simulink model "SLIPquadold"  (R2015a)
settings: Solver=ode45  StartTime=0.0  StopTime=5  MaxStep=1e-3  RelTol=1e-4  AbsTol=1e-6
values from neighbouring files (symbols this model uses):
  a0 = 68*pi/180    (= 1.18682389136)    [smm_params.m]
  dt0 = -0.3325    [SLIPquad_params.m]
  dx0 = 0.4138    [SLIPquad_params.m]    (also in SLIPrun_params.m = 3; SLIPwalk_params.m = 2.5; smm_params.m = 5)
  dy0 = 0.1683    [SLIPquad_params.m]    (also in SLIPrun_params.m = -1; SLIPwalk_params.m = 0; smm_params.m = 0)
  g = 1    [SLIPquad_params.m]    (also in SLIPrun_params.m = 9.81; SLIPwalk_params.m = 9.81; smm_params.m = 9.81)
  J = 0.6    [SLIPquad_params.m]
  k = 20    [SLIPquad_params.m]    (also in SLIPrun_params.m = 23000; SLIPwalk_params.m = 10000; smm_params.m = 20000)
  L = sqrt( (u(3)-u(1))^2 + (u(4)-u(2))^2 )    [AnimSMR.m]    (also in SLIPquad_params.m = 0.5)
  l0 = 1    [SLIPquad_params.m]    (also in SLIPrun_params.m; SLIPwalk_params.m; smm_params.m)
  m = 1    [SLIPquad_params.m]    (also in SLIPrun_params.m = 70; SLIPwalk_params.m = 70; smm_params.m = 80)
  t0 = 0.056    [SLIPquad_params.m]
  x0 = []    [AnimQUAD.m]    (also in AnimQUAD2.m; AnimSMR.m; SLIPquad_params.m = 0; SLIPrun_params.m = -l*sin(theta_th))
  xrb0 = -l0*cos(a0br) + L*cos(t0)    [SLIPquad_params.m]
  xrf0 = -l0*cos(a0fr) - L*cos(t0)    [SLIPquad_params.m]
  y0 = 1.0237    [SLIPquad_params.m]    (also in SLIPrun_params.m = sqrt(l^2 - x0^2); SLIPwalk_params.m = sqrt(l0^2 - x0^2); smm_params.m = 1)
  yrb0 = l0*sin(a0br) + L*sin(t0)    [SLIPquad_params.m]
  yrf0 = l0*sin(a0fr) - L*sin(t0)    [SLIPquad_params.m]
libraries: simulink_extras x2
settings Model: Creator=hgeyer  LastModifiedBy=Joe
settings DataIOCC: LimitDataPoints=off  SignalLoggingSaveFormat=ModelDataLogs
settings OptimizationCC: ExpressionDepthLimit=2147483647
settings DebuggingCC: UnderspecifiedInitializationDetection=Classic  MergeDetectMultiDrivingBlocksExec=none  SolverPrmCheckMsg=warning  FcnCallInpInsideContextMsg=EnableAllAsWarning  StateNameClashWarn=warning

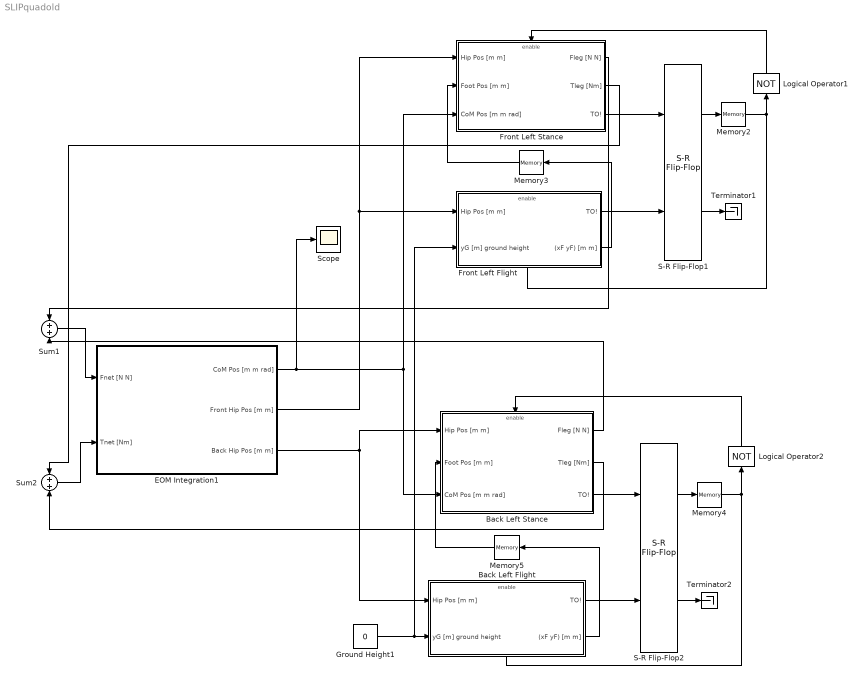
== system SLIPquadold ==
  Back Left Flight : Subsystem
  Back Left Stance : Subsystem
  EOM Integration1 : Subsystem
  Front Left Flight : Subsystem
  Front Left Stance : Subsystem
  Ground Height1 : Constant  Value=0
  Logical Operator1 : Logic  Operator=NOT  AllPortsSameDT=off  OutDataTypeStr=boolean
  Logical Operator2 : Logic  Operator=NOT  AllPortsSameDT=off  OutDataTypeStr=boolean
  Memory2 : Memory  X0=1
  Memory3 : Memory  X0=[(x0 - xrf0) (y0 - yrf0)]
  Memory4 : Memory  X0=1
  Memory5 : Memory  X0=[(x0 - xrb0) (y0 - yrb0)]
  S-R Flip-Flop1 : simulink_extras/Flip Flops/S-R Flip-Flop  initial_condition=1
  S-R Flip-Flop2 : simulink_extras/Flip Flops/S-R Flip-Flop  initial_condition=1
  Scope : Scope
  Sum1 : Sum  Inputs=+|+
  Sum2 : Sum  Inputs=+|+
  Terminator1 : Terminator
  Terminator2 : Terminator
  wires:
  Front Left Stance/3(TO!) -> S-R Flip-Flop1/1
  S-R Flip-Flop1/1 -> Memory2/1
  Front Left Flight/1(TO!) -> S-R Flip-Flop1/2
  Memory2/1 -> Front Left Flight/Enable, Logical Operator1/1
  Logical Operator1/1 -> Front Left Stance/Enable
  S-R Flip-Flop1/2 -> Terminator1/1
  Front Left Flight/2((xF yF) [m m]) -> Memory3/1
  Memory3/1 -> Front Left Stance/2(Foot Pos [m m])
  Back Left Stance/3(TO!) -> S-R Flip-Flop2/1
  S-R Flip-Flop2/1 -> Memory4/1
  Back Left Flight/1(TO!) -> S-R Flip-Flop2/2
  Memory4/1 -> Back Left Flight/Enable, Logical Operator2/1
  Logical Operator2/1 -> Back Left Stance/Enable
  S-R Flip-Flop2/2 -> Terminator2/1
  Back Left Flight/2((xF yF) [m m]) -> Memory5/1
  Memory5/1 -> Back Left Stance/2(Foot Pos [m m])
  Front Left Stance/1(Fleg [N N]) -> Sum1/1
  Back Left Stance/1(Fleg [N N]) -> Sum1/2
  Front Left Stance/2(Tleg [Nm]) -> Sum2/1
  Back Left Stance/2(Tleg [Nm]) -> Sum2/2
  Sum1/1 -> EOM Integration1/1(Fnet [N N])
  Sum2/1 -> EOM Integration1/2(Tnet [Nm])
  EOM Integration1/2(Front Hip Pos [m m]) -> Front Left Flight/1(Hip Pos [m m]), Front Left Stance/1(Hip Pos [m m])
  EOM Integration1/3(Back Hip Pos [m m]) -> Back Left Flight/1(Hip Pos [m m]), Back Left Stance/1(Hip Pos [m m])
  EOM Integration1/1(CoM Pos [m m rad]) -> Scope/1, Front Left Stance/3(CoM Pos [m m rad]), Back Left Stance/3(CoM Pos [m m rad])
  Ground Height1/1 -> Front Left Flight/2(yG [m] ground height), Back Left Flight/2(yG [m] ground height)

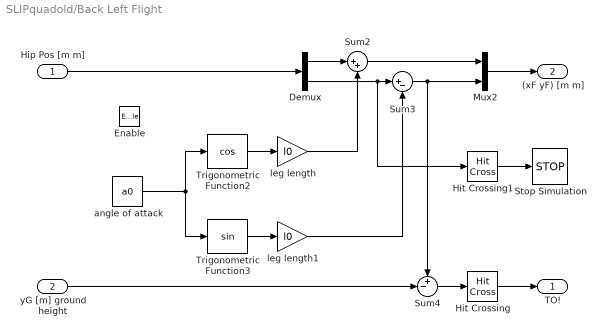
== system SLIPquadold/Back Left Flight ==
  Hip Pos [m m] : Inport
  yG [m] ground height : Inport  Port=2
  Enable : EnablePort  StatesWhenEnabling=reset
  Demux : Demux  Outputs=2
  Hit Crossing : HitCross  HitCrossingDirection=falling
  Hit Crossing1 : HitCross  HitCrossingDirection=falling
  Mux2 : Mux  Inputs=2
  Stop Simulation : Stop
  Sum2 : Sum  Inputs=|++
  Sum3 : Sum  Inputs=|+-
  Sum4 : Sum  Inputs=+-|
  Trigonometric Function2 : Trigonometry  Operator=cos
  Trigonometric Function3 : Trigonometry
  angle of attack : Constant  Value=a0
  leg length : Gain  Gain=l0
  leg length1 : Gain  Gain=l0
  TO! : Outport  OutputWhenDisabled=reset  InitialOutput=0
      settings: AttributesFormatString=%<OutputWhenDisabled>
  (xF yF) [m m] : Outport  Port=2  InitialOutput=[0 0]
      settings: AttributesFormatString=%<OutputWhenDisabled>
  wires:
  Hit Crossing/1 -> TO!/1
  Demux/2 -> Hit Crossing1/1, Sum3/1
  Demux/1 -> Sum2/1
  angle of attack/1 -> Trigonometric Function3/1, Trigonometric Function2/1
  Trigonometric Function2/1 -> leg length/1
  Trigonometric Function3/1 -> leg length1/1
  Hip Pos [m m]/1 -> Demux/1
  leg length/1 -> Sum2/2
  leg length1/1 -> Sum3/2
  Sum3/1 -> Mux2/2, Sum4/1
  Sum2/1 -> Mux2/1
  Mux2/1 -> (xF yF) [m m]/1
  yG [m] ground height/1 -> Sum4/2
  Sum4/1 -> Hit Crossing/1
  Hit Crossing1/1 -> Stop Simulation/1

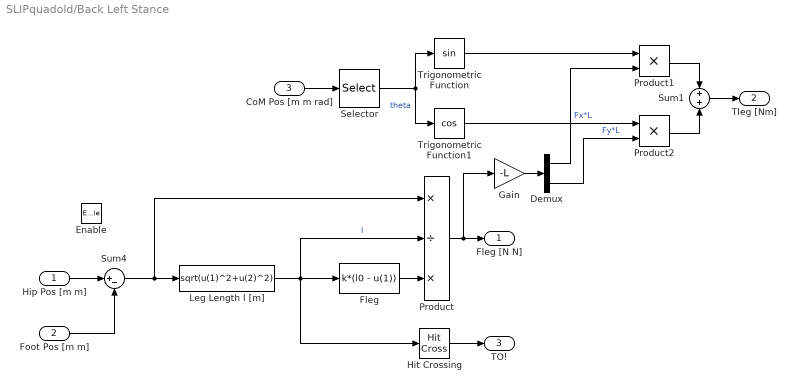
== system SLIPquadold/Back Left Stance ==
  Hip Pos [m m] : Inport
  Foot Pos [m m] : Inport  Port=2
  CoM Pos [m m rad] : Inport  Port=3
  Enable : EnablePort  StatesWhenEnabling=reset
  Demux : Demux  Outputs=2
  Fleg : Fcn  Expr=k*(l0 - u(1))
  Gain : Gain  Gain=-L
  Hit Crossing : HitCross  HitCrossingOffset=l0  HitCrossingDirection=rising
  Leg Length l [m] : Fcn  Expr=sqrt(u(1)^2+u(2)^2)
  Product : Product  Inputs=*/*
  Product1 : Product
  Product2 : Product
  Selector : Selector  InputPortWidth=3  Indices=[3]
  Sum1 : Sum  Inputs=+|+
  Sum4 : Sum  Inputs=|+-
  Trigonometric Function : Trigonometry
  Trigonometric Function1 : Trigonometry  Operator=cos
  Fleg [N N] : Outport  OutputWhenDisabled=reset  InitialOutput=[0 0]
      settings: AttributesFormatString=%<OutputWhenDisabled>
  Tleg [Nm] : Outport  Port=2  OutputWhenDisabled=reset  InitialOutput=[0]
      settings: AttributesFormatString=%<OutputWhenDisabled>
  TO! : Outport  Port=3  OutputWhenDisabled=reset  InitialOutput=[0]
      settings: AttributesFormatString=%<OutputWhenDisabled>
  wires:
  Sum1/1 -> Tleg [Nm]/1
  Product1/1 -> Sum1/1
  Product2/1 -> Sum1/2
  Gain/1 -> Demux/1
  Demux/2 -> Product2/2  "Fy*L"
  Demux/1 -> Product1/2  "Fx*L"
  Trigonometric Function/1 -> Product1/1
  Trigonometric Function1/1 -> Product2/1
  Selector/1 -> Trigonometric Function/1, Trigonometric Function1/1  "theta"
  CoM Pos [m m rad]/1 -> Selector/1
  Foot Pos [m m]/1 -> Sum4/2
  Hip Pos [m m]/1 -> Sum4/1
  Hit Crossing/1 -> TO!/1
  Product/1 -> Fleg [N N]/1, Gain/1
  Fleg/1 -> Product/3
  Leg Length l [m]/1 -> Hit Crossing/1, Product/2, Fleg/1  "l"
  Sum4/1 -> Leg Length l [m]/1, Product/1

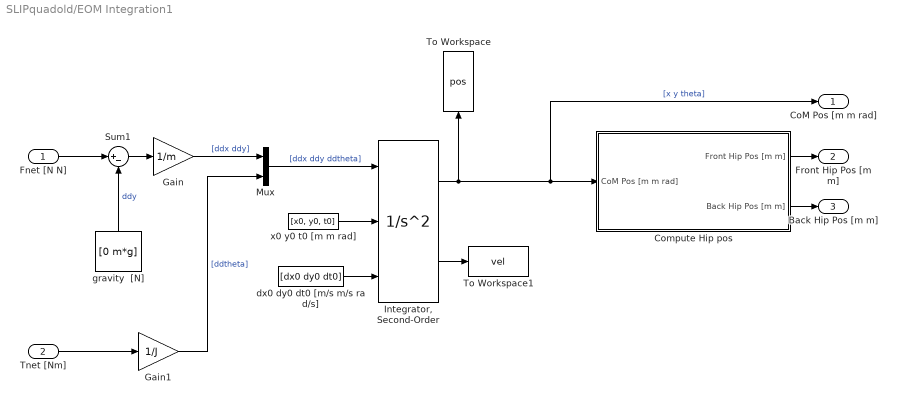
== system SLIPquadold/EOM Integration1 ==
  Fnet [N N] : Inport
  Tnet [Nm] : Inport  Port=2
  Compute Hip pos : Subsystem
  Gain : Gain  Gain=1/m
  Gain1 : Gain  Gain=1/J
  "Integrator, Second-Order" : SecondOrderIntegrator  ICSourceX=external  ICSourceDXDT=external
  Mux : Mux  Inputs=2
  Sum1 : Sum  Inputs=|+-
  To Workspace : ToWorkspace  VariableName=pos  SampleTime=-1
  To Workspace1 : ToWorkspace  VariableName=vel  SampleTime=-1
  dx0 dy0 dt0 [m/s m/s ra d/s] : Constant  Value=[dx0 dy0 dt0]
  gravity  [N] : Constant  Value=[0 m*g]
  x0 y0 t0 [m m rad] : Constant  Value=[x0, y0, t0]
  CoM Pos [m m rad] : Outport
  Front Hip Pos [m m] : Outport  Port=2
  Back Hip Pos [m m] : Outport  Port=3
  wires:
  "Integrator, Second-Order"/2 -> To Workspace1/1
  Compute Hip pos/1(Front Hip Pos [m m]) -> Front Hip Pos [m m]/1
  "Integrator, Second-Order"/1 -> To Workspace/1, CoM Pos [m m rad]/1, Compute Hip pos/1(CoM Pos [m m rad])  "[x y theta]"
  Tnet [Nm]/1 -> Gain1/1
  Gain1/1 -> Mux/2  "[ddtheta]"
  Mux/1 -> "Integrator, Second-Order"/1  "[ddx ddy ddtheta]"
  dx0 dy0 dt0 [m/s m/s ra d/s]/1 -> "Integrator, Second-Order"/3
  Fnet [N N]/1 -> Sum1/1
  Gain/1 -> Mux/1  "[ddx ddy]"
  x0 y0 t0 [m m rad]/1 -> "Integrator, Second-Order"/2
  gravity  [N]/1 -> Sum1/2  "ddy"
  Sum1/1 -> Gain/1
  Compute Hip pos/2(Back Hip Pos [m m]) -> Back Hip Pos [m m]/1

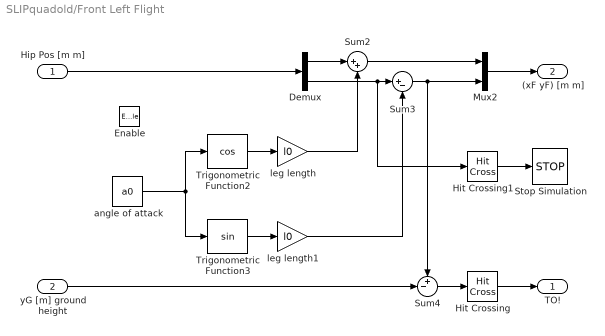
== system SLIPquadold/Front Left Flight ==
  Hip Pos [m m] : Inport
  yG [m] ground height : Inport  Port=2
  Enable : EnablePort  StatesWhenEnabling=reset
  Demux : Demux  Outputs=2
  Hit Crossing : HitCross  HitCrossingDirection=falling
  Hit Crossing1 : HitCross  HitCrossingDirection=falling
  Mux2 : Mux  Inputs=2
  Stop Simulation : Stop
  Sum2 : Sum  Inputs=|++
  Sum3 : Sum  Inputs=|+-
  Sum4 : Sum  Inputs=+-|
  Trigonometric Function2 : Trigonometry  Operator=cos
  Trigonometric Function3 : Trigonometry
  angle of attack : Constant  Value=a0
  leg length : Gain  Gain=l0
  leg length1 : Gain  Gain=l0
  TO! : Outport  OutputWhenDisabled=reset  InitialOutput=0
      settings: AttributesFormatString=%<OutputWhenDisabled>
  (xF yF) [m m] : Outport  Port=2  InitialOutput=[0 0]
      settings: AttributesFormatString=%<OutputWhenDisabled>
  wires:
  Hit Crossing1/1 -> Stop Simulation/1
  Sum4/1 -> Hit Crossing/1
  yG [m] ground height/1 -> Sum4/2
  Mux2/1 -> (xF yF) [m m]/1
  Sum2/1 -> Mux2/1
  Sum3/1 -> Sum4/1, Mux2/2
  leg length1/1 -> Sum3/2
  leg length/1 -> Sum2/2
  Hip Pos [m m]/1 -> Demux/1
  Trigonometric Function3/1 -> leg length1/1
  Trigonometric Function2/1 -> leg length/1
  angle of attack/1 -> Trigonometric Function2/1, Trigonometric Function3/1
  Demux/1 -> Sum2/1
  Demux/2 -> Sum3/1, Hit Crossing1/1
  Hit Crossing/1 -> TO!/1

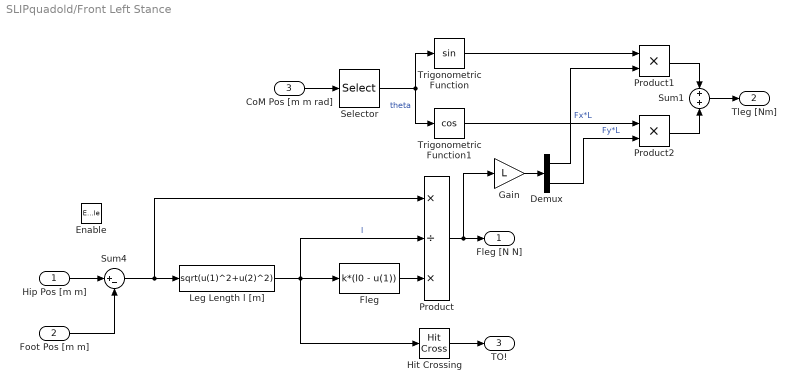
== system SLIPquadold/Front Left Stance ==
  Hip Pos [m m] : Inport
  Foot Pos [m m] : Inport  Port=2
  CoM Pos [m m rad] : Inport  Port=3
  Enable : EnablePort  StatesWhenEnabling=reset
  Demux : Demux  Outputs=2
  Fleg : Fcn  Expr=k*(l0 - u(1))
  Gain : Gain  Gain=L
  Hit Crossing : HitCross  HitCrossingOffset=l0  HitCrossingDirection=rising
  Leg Length l [m] : Fcn  Expr=sqrt(u(1)^2+u(2)^2)
  Product : Product  Inputs=*/*
  Product1 : Product
  Product2 : Product
  Selector : Selector  InputPortWidth=3  Indices=[3]
  Sum1 : Sum  Inputs=+|+
  Sum4 : Sum  Inputs=|+-
  Trigonometric Function : Trigonometry
  Trigonometric Function1 : Trigonometry  Operator=cos
  Fleg [N N] : Outport  OutputWhenDisabled=reset  InitialOutput=[0 0]
      settings: AttributesFormatString=%<OutputWhenDisabled>
  Tleg [Nm] : Outport  Port=2  OutputWhenDisabled=reset  InitialOutput=[0]
      settings: AttributesFormatString=%<OutputWhenDisabled>
  TO! : Outport  Port=3  OutputWhenDisabled=reset  InitialOutput=[0]
      settings: AttributesFormatString=%<OutputWhenDisabled>
  wires:
  Sum4/1 -> Product/1, Leg Length l [m]/1
  Leg Length l [m]/1 -> Fleg/1, Product/2, Hit Crossing/1  "l"
  Fleg/1 -> Product/3
  Product/1 -> Gain/1, Fleg [N N]/1
  Hit Crossing/1 -> TO!/1
  Hip Pos [m m]/1 -> Sum4/1
  Foot Pos [m m]/1 -> Sum4/2
  CoM Pos [m m rad]/1 -> Selector/1
  Selector/1 -> Trigonometric Function1/1, Trigonometric Function/1  "theta"
  Trigonometric Function1/1 -> Product2/1
  Trigonometric Function/1 -> Product1/1
  Demux/1 -> Product1/2  "Fx*L"
  Demux/2 -> Product2/2  "Fy*L"
  Gain/1 -> Demux/1
  Product2/1 -> Sum1/2
  Product1/1 -> Sum1/1
  Sum1/1 -> Tleg [Nm]/1

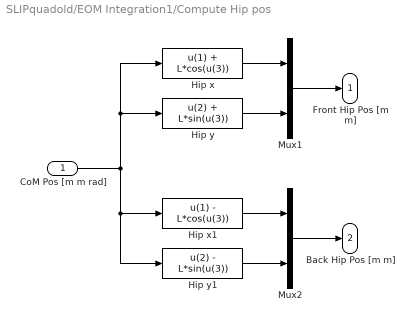
== system SLIPquadold/EOM Integration1/Compute Hip pos ==
  CoM Pos [m m rad] : Inport
  Hip x : Fcn  Expr=u(1) + L*cos(u(3))
  Hip x1 : Fcn  Expr=u(1) - L*cos(u(3))
  Hip y : Fcn  Expr=u(2) + L*sin(u(3))
  Hip y1 : Fcn  Expr=u(2) - L*sin(u(3))
  Mux1 : Mux  Inputs=2
  Mux2 : Mux  Inputs=2
  Front Hip Pos [m m] : Outport
  Back Hip Pos [m m] : Outport  Port=2
  wires:
  Hip y/1 -> Mux1/2
  Mux1/1 -> Front Hip Pos [m m]/1
  Hip x/1 -> Mux1/1
  Hip y1/1 -> Mux2/2
  Mux2/1 -> Back Hip Pos [m m]/1
  Hip x1/1 -> Mux2/1
  CoM Pos [m m rad]/1 -> Hip x/1, Hip y/1, Hip y1/1, Hip x1/1
